simulink model "IntentoDeSimulacionCompletaSimulink"  (R2018a)
settings: Solver=VariableStepAuto  StartTime=0.0  StopTime=10.0  RelTol=1e-3
values from neighbouring files (symbols this model uses):
  F = 1.015    [IntentoDeSimulacionCompletaSimulink.m]    (also in calculo_de_F.m = (1-Kp)/Kp)
  Gextcircuito = -50/((s/0.1)+1)    [IntentoDeSimulacionCompletaSimulink.m]
settings Model: Creator=Ignacio  LastModifiedBy=Ignacio

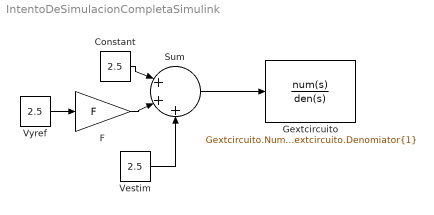
== system IntentoDeSimulacionCompletaSimulink ==
  Constant : Constant  Value=2.5
  F : Gain  Gain=F
  Gextcircuito : TransferFcn  Numerator=Gextcircuito.Numerator{1}  Denominator=Gextcircuito.Denomiator{1}
  Sum : Sum  Inputs=|+++
  Vestim : Constant  Value=2.5
  Vyref : Constant  Value=2.5
  wires:
  F/1 -> Sum/2
  Constant/1 -> Sum/1
  Vyref/1 -> F/1
  Vestim/1 -> Sum/3
  Sum/1 -> Gextcircuito/1
